simulink model "IDRA_mismodeled_A"  (R2024b)
settings: Solver=ode4  StartTime=T_in_sim_A  StopTime=T_sim_A  FixedStep=t_sim  RelTol=1e-3
model workspace (MAT data in the model file):
  A_c = [1; 1; 1; 1; 1]
  A_v = [0.146  0  0  0  0; 0  0.146  0  0  0; 0  0  0.146  0  0; 0  0  0  0.146  0; 0  0  0  0  0.146]
  DELTA = [0.00153398078789; 0.00153398078789; 0.00153398078789; 0.00153398078789; 0.00153398078789]
  K = 5
  Kd = [4  0  0  0  0; 0  4  0  0  0; 0  0  4  0  0; 0  0  0  4  0; 0  0  0  0  4]
  Ki = [28  0  0  0  0; 0  28  0  0  0; 0  0  28  0  0; 0  0  0  28  0; 0  0  0  0  28]
  Kp = [21  0  0  0  0; 0  21  0  0  0; 0  0  21  0  0; 0  0  0  21  0; 0  0  0  0  21]
  M_m = [0.54  0  0  0  0; 0  0.54  0  0  0; 0  0  0.54  0  0; 0  0  0  0.54  0; 0  0  0  0  0.54]
  Ra = [0.103; 0.103; 0.103; 0.103; 0.103]
  T_c = 0.01
  T_gt = 0.005
  T_in_sim_A = 0
  T_in_sim_B = 25.02
  T_moto_A = 9.56
  T_moto_B = 34.085
  T_s = 0.01
  T_sim_A = 25.015
  T_sim_B = 48.735
  T_u = 0.02
  f_c = 50
  f_gt = 200
  f_s = 100
  f_u = 50
  gear_ratio = [100; 100; 100; 100; 100]
  kd = 4
  ke = [0.0385; 0.0385; 0.0385; 0.0385; 0.0385]
  ki = 28
  km = [0.0385; 0.0385; 0.0385; 0.0385; 0.0385]
  kp = 21
  q0_A = [0; -2.4435; 1.5708; 1.5708; 1.5708]
  q0_B = [3.82862160983e-16; -0.562806100915; 2.41996424612; -0.534908886278; 0.248547067871]
  qd0_A = [0; 0; 0; 0; 0]
  qd0_B = [0; 0; 0; 0; 0]
  qdd0_A = [2.20373308525e-17; 0.108251684053; 0.0488774168534; -0.121203420277; -0.0761081357875]
  qdd0_B = [-4.87408370682e-17; 0.121203420277; -0.0531243011007; 0.0781005207217; 0.054950573486]
  t_LPF = 10
  t_const = 0.02
  t_fade = 0.5
  t_sim = 0.005
undefined symbols (not defined in the file or in its folder): DiscIntNeverNeededParam
settings Model: SimulationMode=rapid-accelerator  Creator=marco  LastModifiedBy=marco

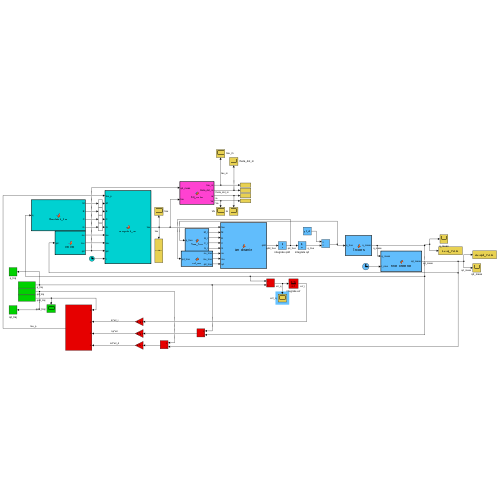
[thumbnail: Simulink's stored preview of the top-level diagram]
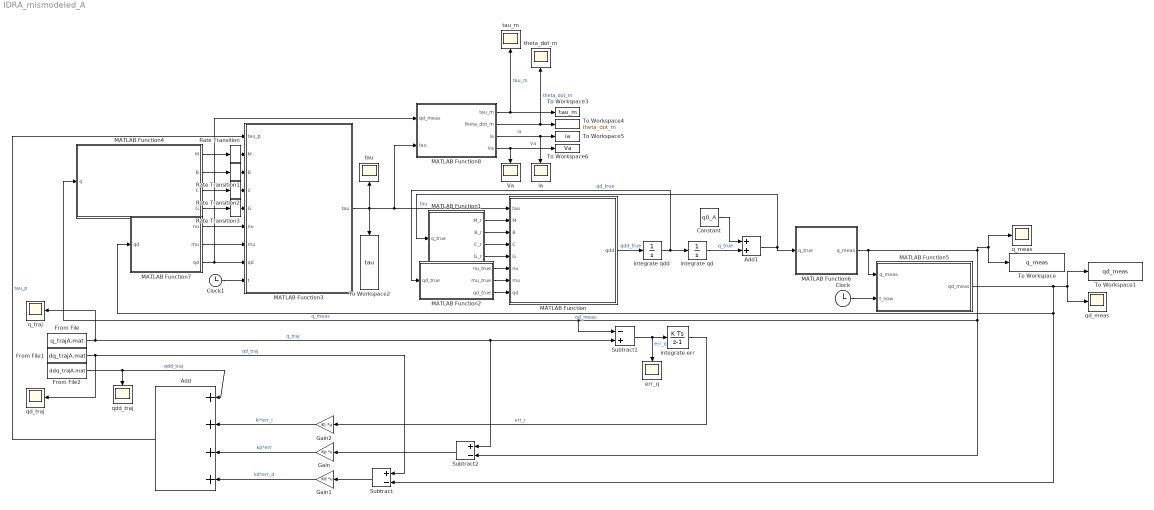
== system IDRA_mismodeled_A ==
  Add : Sum  Inputs=++++
  Add1 : Sum
  Clock : Clock
  Clock1 : Clock
  Constant : Constant  Value=q0_A
  From File : FromFile  FileName=q_trajA.mat  SampleTime=T_gt
  From File1 : FromFile  FileName=dq_trajA.mat  SampleTime=T_gt
  From File2 : FromFile  FileName=ddq_trajA.mat  SampleTime=T_gt
  Gain : Gain  Gain=Kp  Multiplication=Matrix(K*u) (u vector)
  Gain1 : Gain  Gain=Kd  Multiplication=Matrix(K*u) (u vector)
  Gain2 : Gain  Gain=Ki  Multiplication=Matrix(K*u) (u vector)
  MATLAB Function : MATLAB Function  TreatAsAtomicUnit=on
  MATLAB Function1 : MATLAB Function  TreatAsAtomicUnit=on
  MATLAB Function2 : MATLAB Function  TreatAsAtomicUnit=on
  MATLAB Function3 : MATLAB Function  TreatAsAtomicUnit=on  SystemSampleTime=T_c
  MATLAB Function4 : MATLAB Function  TreatAsAtomicUnit=on  SystemSampleTime=T_u
  MATLAB Function5 : MATLAB Function  TreatAsAtomicUnit=on
  MATLAB Function6 : MATLAB Function  TreatAsAtomicUnit=on  SystemSampleTime=T_s
  MATLAB Function7 : MATLAB Function  TreatAsAtomicUnit=on
  MATLAB Function8 : MATLAB Function  TreatAsAtomicUnit=on
  Rate Transition{,1..3} (4 alike) : RateTransition  OutPortSampleTime=T_u
  Subtract : Sum  Inputs=+-
  Subtract1 : Sum  Inputs=-+
  Subtract2 : Sum  Inputs=+-
  To Workspace : ToWorkspace  VariableName=q_meas  SaveFormat=Timeseries  SampleTime=-1
  To Workspace1 : ToWorkspace  VariableName=qd_meas  SaveFormat=Timeseries  SampleTime=-1
  To Workspace2 : ToWorkspace  VariableName=tau  SaveFormat=Timeseries  SampleTime=-1
  To Workspace3 : ToWorkspace  VariableName=tau_m  SaveFormat=Timeseries  SampleTime=-1
  To Workspace4 : ToWorkspace  VariableName=theta_dot_m  SaveFormat=Timeseries  SampleTime=-1
  To Workspace5 : ToWorkspace  VariableName=ia  SaveFormat=Timeseries  SampleTime=-1
  To Workspace6 : ToWorkspace  VariableName=Va  SaveFormat=Timeseries  SampleTime=-1
  Va : Scope
  err_q : Scope
  ia : Scope
  integrate err : DiscreteIntegrator  SampleTime=T_s  ICPrevOutput=DiscIntNeverNeededParam  ICPrevScaledInput=DiscIntNeverNeededParam
  integrate qd : Integrator  InitialCondition=qd0_A
  integrate qdd : Integrator  InitialCondition=qdd0_A
  q_meas : Scope
  q_traj : Scope
  qd_meas : Scope
  qd_traj : Scope
  qdd_traj : Scope
  tau : Scope
  tau_m : Scope
  theta_dot_m : Scope
  wires:
  integrate err/1 -> Gain2/1  "err_i"
  MATLAB Function/1(qdd) -> integrate qdd/1  "qdd_true"
  MATLAB Function1/1(M_r) -> MATLAB Function/2(M)
  MATLAB Function1/2(B_r) -> MATLAB Function/3(B)
  MATLAB Function1/3(C_r) -> MATLAB Function/4(C)
  MATLAB Function1/4(G_r) -> MATLAB Function/5(G)
  MATLAB Function2/1(nu_true) -> MATLAB Function/6(nu)
  MATLAB Function2/2(mu_true) -> MATLAB Function/7(mu)
  MATLAB Function3/1(tau) -> MATLAB Function/1(tau), MATLAB Function8/2(tau), To Workspace2/1, tau/1  "tau"
  Add/1 -> MATLAB Function3/1(tau_p)  "tau_p"
  Subtract1/1 -> err_q/1, integrate err/1  "err_q"
  Subtract2/1 -> Gain/1
  Subtract/1 -> Gain1/1
  From File/1 -> q_traj/1, Subtract2/1, Subtract1/2  "q_traj"
  From File1/1 -> Subtract/1, qd_traj/1  "qd_traj"
  Gain2/1 -> Add/2  "ki*err_i"
  Gain/1 -> Add/3  "kp*err"
  Gain1/1 -> Add/4  "kd*err_d"
  From File2/1 -> qdd_traj/1, Add/1  "qdd_traj"
  MATLAB Function2/3(qd_true) -> MATLAB Function/8(qd)
  integrate qdd/1 -> integrate qd/1, MATLAB Function2/1("qd_true ")  "qd_true"
  MATLAB Function5/1(qd_meas) -> To Workspace1/1, qd_meas/1, MATLAB Function7/1("qd "), Subtract/2  "qd_meas"
  MATLAB Function7/1(nu) -> MATLAB Function3/6(nu)
  MATLAB Function7/2(mu) -> MATLAB Function3/7(mu)
  MATLAB Function7/3(qd) -> MATLAB Function8/1(qd_meas), MATLAB Function3/8(qd)
  MATLAB Function6/1(q_meas) -> MATLAB Function5/1(q_meas), To Workspace/1, q_meas/1, MATLAB Function4/1(q), Subtract1/1, Subtract2/2  "q_meas"
  integrate qd/1 -> Add1/2  "q_true"
  Add1/1 -> MATLAB Function1/1(q_true), MATLAB Function6/1(q_true)
  Constant/1 -> Add1/1
  Clock/1 -> MATLAB Function5/2(t_now)
  Clock1/1 -> MATLAB Function3/9(t)
  MATLAB Function8/1(tau_m) -> tau_m/1, To Workspace3/1  "tau_m"
  MATLAB Function8/2(theta_dot_m) -> theta_dot_m/1, To Workspace4/1  "theta_dot_m"
  MATLAB Function8/3(ia) -> ia/1, To Workspace5/1  "ia"
  MATLAB Function8/4(Va) -> Va/1, To Workspace6/1  "Va"
  Rate Transition/1 -> MATLAB Function3/2(M)
  MATLAB Function4/1(M) -> Rate Transition/1
  Rate Transition1/1 -> MATLAB Function3/3(B)
  MATLAB Function4/2(B) -> Rate Transition1/1
  Rate Transition2/1 -> MATLAB Function3/4(C)
  MATLAB Function4/3(C) -> Rate Transition2/1
  Rate Transition3/1 -> MATLAB Function3/5(G)
  MATLAB Function4/4(G) -> Rate Transition3/1

== matlab function IDRA_mismodeled_A/MATLAB Function7 ==
  data: nu output; mu output; qd input; qd output
function [nu,mu,qd] = vel_vec(qd)
%#codegen
nu = cross_joint_velocity_vector(qd);    % 10x1
mu = squared_joint_velocity_vector(qd);  % 5x1
end

== matlab function IDRA_mismodeled_A/MATLAB Function8 ==
  data: qd_meas input; tau_m output; tau input; theta_dot_m output; ia output; Va output; km parameter; ke parameter; Ra parameter; gear_ratio parameter
function [tau_m,theta_dot_m,ia,Va] = DC_motor(qd_meas,tau,km, ke, Ra, gear_ratio)
%%% function che da modello dei DC Motor

% caratteristiche di lavoro motore
tau_m = tau ./ gear_ratio; % [N*m]
theta_dot_m = qd_meas .* gear_ratio; % [rad/s]
ia = tau_m ./ km; % [A]
Va = Ra .* ia + ke .* theta_dot_m;

== matlab function IDRA_mismodeled_A/MATLAB Function1 ==
  data: q_true input; M_r output; B_r output; C_r output; G_r output
function [M_r,B_r,C_r,G_r] = Real_Arm(q_true)
% M B C G dipendono da modello dinamico
M_r = mass_matrix(q_true);
B_r = cor_coeff_matrix(q_true);
C_r = cent_coeff_matrix(q_true);
G_r = gravity_vector_A(q_true);

end

== matlab function IDRA_mismodeled_A/MATLAB Function ==
  data: tau input; qdd output; M input; B input; C input; G input; nu input; mu input; qd input; M_m parameter double size=[5 5]; A_v parameter double size=[5 5]; A_c parameter double size=[5 1]
function qdd = Arm_dynamics(tau,M,B,C,G,nu,mu,qd, M_m, A_v, A_c)
% tau(dipende da modello dinamica) (M, B, C, G , M_m , A_v , A_c simulano braccio reale)
qdd = (M+M_m) \ (tau - B*nu - C*mu - G - A_v*qd - A_c.*sign(qd));
end

== matlab function IDRA_mismodeled_A/MATLAB Function2 ==
  data: nu_true output; mu_true output; qd_true input; qd_true output
function [nu_true,mu_true,qd_true] = vel_vec(qd_true)
%#codegen
nu_true = cross_joint_velocity_vector(qd_true);    % 10x1
mu_true = squared_joint_velocity_vector(qd_true);  % 5x1
end

== matlab function IDRA_mismodeled_A/MATLAB Function3 ==
  settings: updateMethod=DISCRETE  sampleTime=T_c
  data: tau_p input; tau output; M input; B input; C input; G input; nu input; mu input; qd input; M_m parameter double size=[5 5]; A_v parameter double size=[5 5]; A_c parameter double size=[5 1]; t input; T_moto_A parameter
function tau = computed_tau(tau_p,M,B,C,G,nu,mu,qd, M_m, A_v, A_c,t, T_moto_A)
A = [0;1;1;1;1];
if t > T_moto_A
    A = zeros(5,1);
end
% ricostruzione tau
tau = (M+M_m)*tau_p + G + B*nu + C*mu + A_v*qd + A.*(A_c.* sign(qd));
end

== matlab function IDRA_mismodeled_A/MATLAB Function4 ==
  settings: updateMethod=DISCRETE  sampleTime=T_u
  data: q input; M output; B output; C output; G output
function [M,B,C,G] = Simulated_Arm(q)
% M B C G dipendono da modello dinamico
M = modified_mass_matrix(q);
B = modified_cor_coeff_matrix(q);
C = modified_cent_coeff_matrix(q);
G = modified_gravity_vector_A(q);
end

== matlab function IDRA_mismodeled_A/MATLAB Function5 ==
  settings: updateMethod=DISCRETE  sampleTime=T_s
  data: q_meas input; qd_meas output; T_s parameter; K parameter; t_const parameter; t_now input; t_LPF parameter; t_fade parameter
function qd_meas = finite_difference(q_meas, T_s, K, t_const, t_now, t_LPF, t_fade)
% q_meas: [n x 1] (assoluto quantizzato e già wrappato se serve)
% Output: qd_meas [n x 1]

% forza colonna (evita 1x5 vs 5x1)
q_meas = q_meas(:);
n = size(q_meas,1);

% K almeno 3 (nota: K deve restare costante durante la simulazione,
% altrimenti il buffer cambia dimensione)
if nargin < 3 || isempty(K), K = 5; end
K = max(3, round(K));

% ---- persistent states ----
persistent q_prev_wrap u_prev u_hist y_prev K_prev is_init
if isempty(is_init)
    q_prev_wrap = q_meas;
    u_prev      = q_meas;                         % unwrapped interno
    u_hist      = repmat(u_prev, 1, K);           % buffer [n x K]
    y_prev      = zeros(n,1, 'like', q_meas);      % stato LPF
    K_prev      = K;
    is_init     = true;
end

% reset se dimensioni cambiano o K cambia
if ~isequal(size(q_prev_wrap), size(q_meas)) || K_prev ~= K
    q_prev_wrap = q_meas;
    u_prev      = q_meas;
    u_hist      = repmat(u_prev, 1, K);
    y_prev      = zeros(n,1, 'like', q_meas);
    K_prev      = K;
end

% ---- unwrap incrementale coerente col wrap ----
dq = q_meas - q_prev_wrap;
%dq = atan2(sin(dq), cos(dq));     % delta minimo in (-pi, pi]
u  = u_prev + dq;                 % unwrapped

q_prev_wrap = q_meas;
u_prev      = u;

% ---- aggiorna buffer (shift a sinistra, nuovo in coda) ----
u_hist(:,1:end-1) = u_hist(:,2:end);
u_hist(:,end)     = u;

% ---- stima derivata: LS slope su finestra K (causale) ----
tt = (-(K-1):0) * T_s;        % 1xK  (ATTENZIONE: NON usare "t")
tt = tt - mean(tt);
den = sum(tt.^2);

qd_raw = (u_hist * tt(:)) / den;  % [n x 1]

% ---- LPF 1° ordine su qd_raw ----
if t_const <= 0
    qd_lpf = qd_raw;
else
    a = exp(-T_s / t_const);
    qd_lpf = a .* y_prev + (1 - a) .* qd_raw;
end
y_prev = qd_lpf;

% ---- peso di mix w(t_now) (1=LPF, 0=RAW), fade morbido ----
if t_fade <= 0
    w = double(t_now <= t_LPF);
else
    s = (t_now - t_LPF) / t_fade;   % scalare
    s = min(max(s, 0), 1);
    w = 0.5 * (1 + cos(pi*s));      % 1 -> 0
end

qd_meas = w .* qd_lpf + (1 - w) .* qd_raw;  % sempre [n x 1]

end

== matlab function IDRA_mismodeled_A/MATLAB Function6 ==
  settings: updateMethod=DISCRETE  sampleTime=T_s
  data: q_true input; q_meas output; DELTA parameter double size=[5 1]; gear_ratio parameter double size=[5 1]
function q_meas  = Encoders(q_true, DELTA, gear_ratio)

    % Encoder assoluto: wrap -> quantize 
    
    % Parametri dal base workspace / model workspace:
    %   DELTA : [nx1] oppure scalar (step quantizzazione [rad])
    
    % ---- wrap q_true in [-pi, pi] ----
    q_true = wrapTo2Pi(q_true);
    % ---- trasforma in q motore
    q_true = q_true .* gear_ratio;
    
    % ---- quantizzazione ----
    q_meas = DELTA .* floor(q_true ./ DELTA); % nella realtà ha piu senso wrappare in [0,2pi] e poi usare floor ma così è piu pulito per controllo

    %----- trasforma in q giunto
    q_meas = wrapToPi(q_meas ./ gear_ratio);
    
  
end
